simulink model "dual_port_ram_interface"  (R2020b)
settings: Solver=FixedStepDiscrete  StartTime=0.0  StopTime=stopTime  RelTol=1e-3
values from neighbouring files (symbols this model uses):
  addr_bits = 16    [modelparameters.m]
libraries: hdlsllib x2
settings Model: Creator=Ross  LastModifiedBy=tyler
settings DataIOCC: SaveOutput=off  SaveTime=off  ReturnWorkspaceOutputs=off
settings OptimizationCC: BlockReduction=off  ConditionallyExecuteInputs=off  DefaultParameterBehavior=Inlined
settings DebuggingCC: ReadBeforeWriteMsg=DisableAll  WriteAfterWriteMsg=DisableAll  WriteAfterReadMsg=DisableAll  AlgebraicLoopMsg=error  MultiTaskDSMMsg=none  SingleTaskRateTransMsg=error  PregeneratedLibrarySubsystemCodeDiagnostic=none  ArithmeticOperatorsInVariantConditions=warning
settings HardwareCC: ProdBitPerPointer=32  ProdBitPerSizeT=32  ProdBitPerPtrDiffT=32  ProdLargestAtomicFloat=None  ProdIntDivRoundTo=Undefined  ProdEndianess=Unspecified  ProdWordSize=32  ProdHWDeviceType=ASIC/FPGA->ASIC/FPGA  TargetBitPerPointer=64  TargetBitPerSizeT=64  TargetBitPerPtrDiffT=64  TargetLongLongMode=on  TargetIntDivRoundTo=Zero  TargetEndianess=LittleEndian  TargetWordSize=64  TargetHWDeviceType=Custom Processor->MATLAB Host Computer  ProdEqTarget=off
settings ModelReferenceCC: UpdateModelReferenceTargets=IfOutOfDate
settings SFSimCC: SFSimEcho=off  SimUseLocalCustomCode=off  CustomCodeUndefinedFunction=UseInterfaceOnly
settings RTWCC: RTWUseLocalCustomCode=off

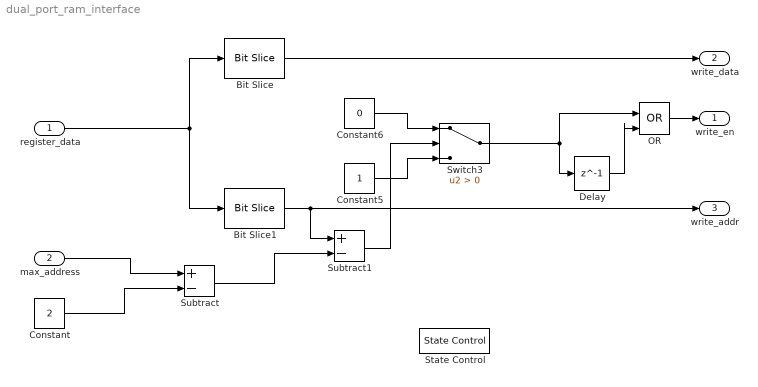
== system dual_port_ram_interface ==
  register_data : Inport  OutDataTypeStr=uint32  PortDimensions=1
  max_address : Inport  Port=2  OutDataTypeStr=uint32  PortDimensions=1
  Bit Slice : hdlsllib/Logic and Bit Operations/Bit Slice  lidx=addr_bits-1  ridx=0
      settings: SourceProductBaseCode=SL
  Bit Slice1 : hdlsllib/Logic and Bit Operations/Bit Slice  lidx=31  ridx=addr_bits
      settings: SourceProductBaseCode=SL
  Constant : Constant  Value=2  OutDataTypeStr=uint8  SampleTime=-1
  Constant5 : Constant  OutDataTypeStr=boolean  SampleTime=-1
  Constant6 : Constant  Value=0  OutDataTypeStr=boolean  SampleTime=-1
  Delay : Delay  DelayLength=1
  OR : Logic  Operator=OR  IconShape=distinctive  AllPortsSameDT=off  OutDataTypeStr=boolean
  State Control : StateControl  StateControl=Synchronous
  Subtract : Sum  Inputs=+-
  Subtract1 : Sum  Inputs=+-  OutDataTypeStr=int8  SaturateOnIntegerOverflow=on
  Switch3 : Switch  Criteria=u2 > Threshold  OutDataTypeStr=boolean
  write_en : Outport  PortDimensions=1
  write_data : Outport  Port=2  OutDataTypeStr=uint16  PortDimensions=1
  write_addr : Outport  Port=3  OutDataTypeStr=uint16  PortDimensions=1
  wires:
  OR/1 -> write_en/1
  Switch3/1 -> OR/1, Delay/1
  Constant6/1 -> Switch3/1
  Constant5/1 -> Switch3/3
  Delay/1 -> OR/2
  register_data/1 -> Bit Slice1/1, Bit Slice/1
  Bit Slice/1 -> write_data/1
  Bit Slice1/1 -> Subtract1/1, write_addr/1
  Constant/1 -> Subtract/2
  max_address/1 -> Subtract/1
  Subtract1/1 -> Switch3/2
  Subtract/1 -> Subtract1/2
